simulink model "TUUM1_Quanser"  (R2021b)
settings: Solver=ode1  StartTime=0.0  StopTime=Tsim  FixedStep=Ts  RelTol=1e-3
InitFcn:
  | Ts=1e-3;  % vrijeme uzorkovanja
  | Tsim = 14.9;  % trajanje eksperimenta, treba završiti dok je referenca 0
  | TUUM1;  % inicijalizacijska skripta
values from neighbouring files (symbols this model uses):
  REF = 5    [TUUM1.m]
undefined symbols (not defined in the file or in its folder): Model_626, Sensoray
libraries: sldrtlib x2
settings Model: SimulationMode=external  Creator=Melab1Guest  LastModifiedBy=Melab1Guest
settings RTWCC: Description=Simulink Desktop Real-Time  SystemTargetFile=sldrt.tlc  TemplateMakefile=sldrt.tmf  RTWCompilerOptimization=on
settings CodeAppCC: MaxIdLength=95
settings SimulinkDesktopRealTimeCC: TargetPreCompLibLocation=C:\Program Files\MATLAB\R2021b\toolbox\sldrt\lib\win64

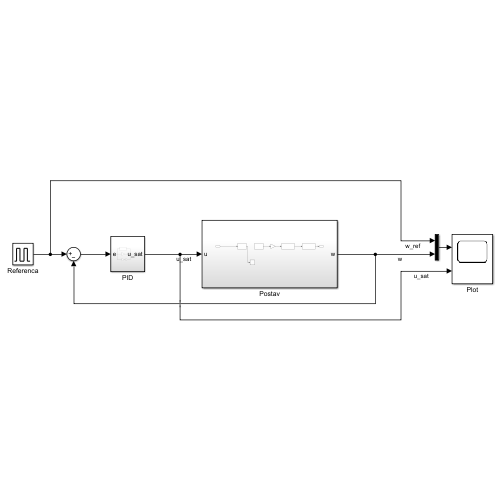
[thumbnail: Simulink's stored preview of the top-level diagram]
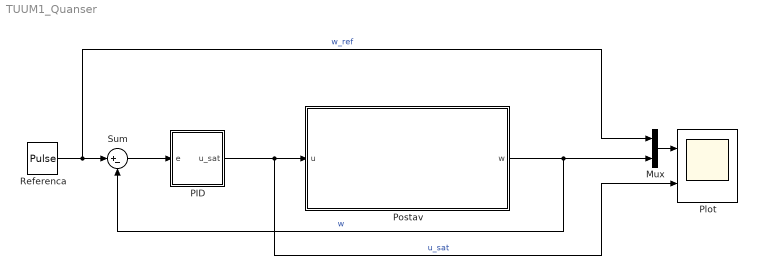
== system TUUM1_Quanser ==
  Mux : Mux  Inputs=2
  PID : Subsystem
  Plot : Scope  NumInputPorts=2
  Postav : Subsystem
  Referenca : DiscretePulseGenerator  PulseType=Time based  Amplitude=REF  Period=5  PulseWidth=50
  Sum : Sum  Inputs=|+-
  wires:
  Postav/1(w) -> Mux/2, Sum/2  "w"
  Referenca/1 -> Mux/1, Sum/1  "w_ref"
  Sum/1 -> PID/1(e)
  Mux/1 -> Plot/1
  PID/1(u_sat) -> Plot/2, Postav/1(u)  "u_sat"

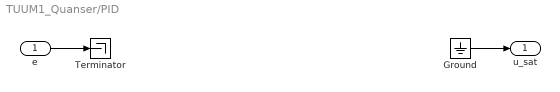
== system TUUM1_Quanser/PID ==
  e : Inport
  Ground : Ground
  Terminator : Terminator
  u_sat : Outport
  wires:
  e/1 -> Terminator/1
  Ground/1 -> u_sat/1

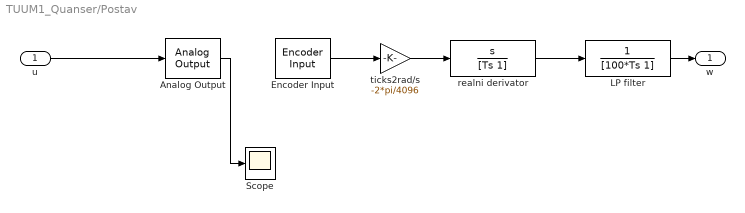
== system TUUM1_Quanser/Postav ==
  u : Inport
  Analog Output : sldrtlib/Analog Output  SampleTime=Ts  MaxMissedTicks=100  ShowMissedTicks=on  YieldWhenWaiting=off  DrvName=Sensoray/Model_626  DrvAddress=4294967295  DrvOptions=zeros(1,0)  Channels=1  RangeMode=1  VoltRange=1  InitialValue=0  FinalValue=0
      settings: AttributesFormatString=Sensoray\nModel 626 [auto]
  Encoder Input : sldrtlib/Encoder Input  SampleTime=Ts  MaxMissedTicks=100  ShowMissedTicks=off  YieldWhenWaiting=off  DrvName=Sensoray/Model_626  DrvAddress=4294967295  DrvOptions=zeros(1,0)  Channels=1  QuadMode=3  IndexPulse=2  InputFilter=Inf  DataType=1
      settings: AttributesFormatString=Sensoray\nModel 626 [auto]
  LP filter : TransferFcn  Denominator=[100*Ts 1]
  Scope : Scope
  realni derivator : TransferFcn  Numerator=[1 0]  Denominator=[Ts 1]
  ticks2rad/s : Gain  Gain=-2*pi/4096
  w : Outport
  wires:
  Encoder Input/1 -> ticks2rad/s/1
  ticks2rad/s/1 -> realni derivator/1
  Analog Output/1 -> Scope/1
  realni derivator/1 -> LP filter/1
  LP filter/1 -> w/1
  u/1 -> Analog Output/1
